simulink model "lab1_system5"  (R2024a)
settings: Solver=VariableStepAuto  StartTime=0.0  StopTime=10.0  RelTol=1e-3
settings Model: Creator=alexivanov  LastModifiedBy=alexivanov

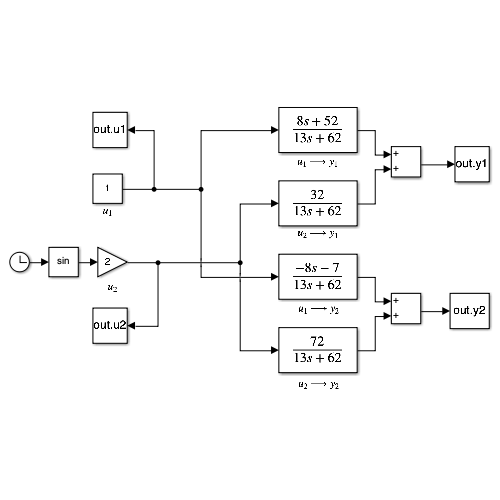
[thumbnail: Simulink's stored preview of the top-level diagram]
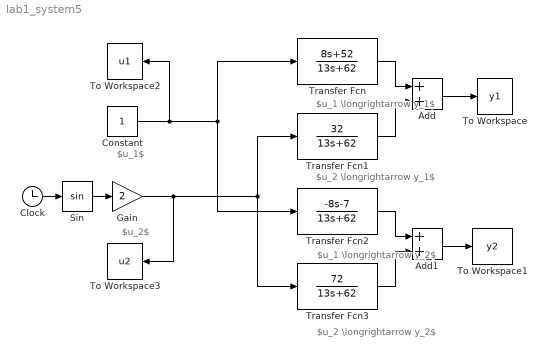
== system lab1_system5 ==
  note: $u_1$
  note: $u_2$
  note: $u_1 \longrightarrow y_1$
  note: $u_2 \longrightarrow y_1$
  note: $u_1 \longrightarrow y_2$
  note: $u_2 \longrightarrow y_2$
  Add : Sum
  Add1 : Sum
  Clock : Clock
  Constant : Constant  SampleTime=0
  Gain : Gain  Gain=2
  Sin : Trigonometry
  To Workspace : ToWorkspace  VariableName=y1  SaveFormat=Timeseries  SampleTime=-1
  To Workspace1 : ToWorkspace  VariableName=y2  SaveFormat=Timeseries  SampleTime=-1
  To Workspace2 : ToWorkspace  VariableName=u1  SaveFormat=Timeseries  SampleTime=-1
  To Workspace3 : ToWorkspace  VariableName=u2  SaveFormat=Timeseries  SampleTime=-1
  Transfer Fcn : TransferFcn  Numerator=[8 52]  Denominator=[13 62]
  Transfer Fcn1 : TransferFcn  Numerator=[32]  Denominator=[13 62]
  Transfer Fcn2 : TransferFcn  Numerator=[-8 -7]  Denominator=[13 62]
  Transfer Fcn3 : TransferFcn  Numerator=[72]  Denominator=[13 62]
  wires:
  Clock/1 -> Sin/1
  Sin/1 -> Gain/1
  Add/1 -> To Workspace/1
  Transfer Fcn/1 -> Add/1
  Transfer Fcn1/1 -> Add/2
  Transfer Fcn2/1 -> Add1/1
  Transfer Fcn3/1 -> Add1/2
  Add1/1 -> To Workspace1/1
  Constant/1 -> To Workspace2/1, Transfer Fcn2/1, Transfer Fcn/1
  Gain/1 -> To Workspace3/1, Transfer Fcn3/1, Transfer Fcn1/1
